simulink model "rlAgentLCLongLat"  (R2024a)
settings: Solver=VariableStepAuto  StartTime=0.0  StopTime=Tf  FixedStep=1e-3  MaxStep=0.1  RelTol=1e-3
values from neighbouring files (symbols this model uses):
  A = [ ... (first row only)    [rlAgentLCParams.m]
  B = [0 2*Cf/m 0 2*lf*Cf/Iz]'    [rlAgentLCParams.m]
  Cf = 19000    [multiAgentPFCParams.m]    (also in rlAgentLCParams.m = 151000)
  Cr = 33000    [multiAgentPFCParams.m]    (also in rlAgentLCParams.m = 146000)
  Iz = 2875    [multiAgentPFCParams.m]    (also in rlAgentLCParams.m = 1993)
  lf = 1.4    [multiAgentPFCParams.m]    (also in rlAgentLCParams.m = 1.45)
  lr = 1.6    [multiAgentPFCParams.m]    (also in rlAgentLCParams.m = 1.06)
  m = 1600    [multiAgentPFCParams.m]    (also in rlAgentLCParams.m = 1360)
  Qlat = diag([20 50 2000 3000])    [rlAgentLCParams.m]
  Rlat = eye(1)    [rlAgentLCParams.m]
  Ts = 0.1    [rlAgentLCParams.m]
  Vx = 20    [rlAgentLCParams.m]
undefined symbols (not defined in the file or in its folder): Qlong, Rlong
libraries: rllib x2, matrix_library x2
settings Model: Creator=The MathWorks, Inc.  LastModifiedBy=canlab
settings SolverCC: AlgebraicLoopSolver=TrustRegion
settings DataIOCC: SaveOutput=off  SignalLogging=off  DSMLogging=off  SaveTime=off  ReturnWorkspaceOutputs=off
settings DebuggingCC: ParameterPrecisionLossMsg=none  UnconnectedInputMsg=warning  UnconnectedOutputMsg=warning  UnconnectedLineMsg=warning  ArithmeticOperatorsInVariantConditions=warning
settings ModelReferenceCC: EnableRefExpFcnMdlSchedulingChecks=on
settings SFSimCC: SimUseLocalCustomCode=off
settings RTWCC: RTWUseLocalCustomCode=off  GPUComputeCapability=3.5  DLArmComputeVersion=19.05

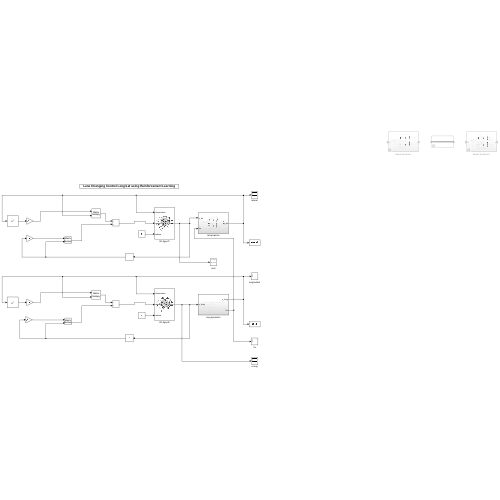
[thumbnail: Simulink's stored preview of the top-level diagram]
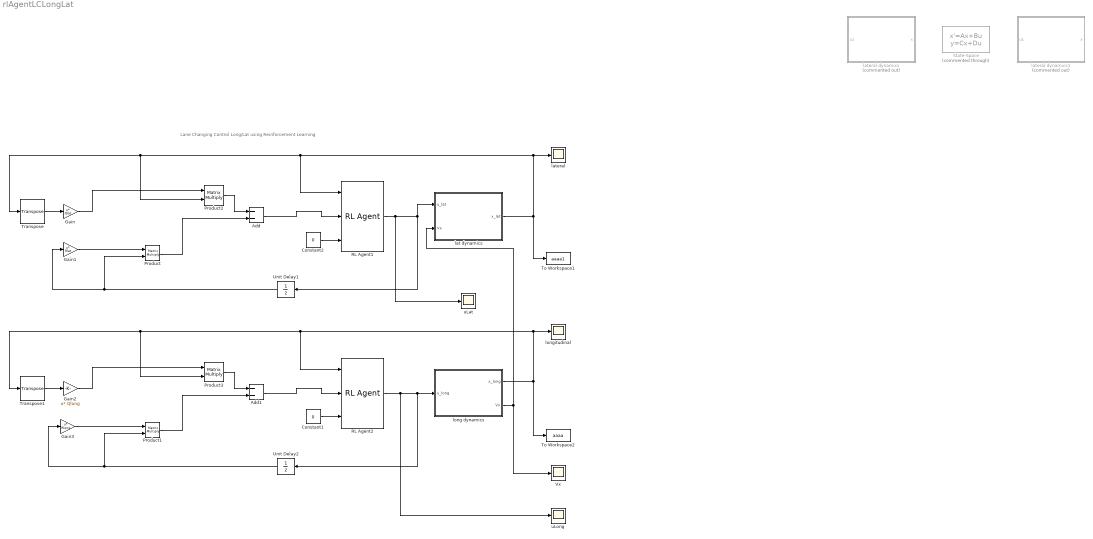
== system rlAgentLCLongLat ==
  note: Lane Changing Control Long/Lat using Reinforcement Learning
  Add : Sum  Inputs=--
  Add1 : Sum  Inputs=--
  Constant1 : Constant  Value=0  SampleTime=Ts
  Constant2 : Constant  Value=0  SampleTime=Ts
  Gain : Gain  Gain=Qlat  Multiplication=Matrix(u*K)
  Gain1 : Gain  Gain=Rlat  Multiplication=Matrix(u*K)
  Gain2 : Gain  Gain=Qlong  Multiplication=Matrix(u*K)
  Gain3 : Gain  Gain=Rlong  Multiplication=Matrix(u*K)
  Product{,1..3} (4 alike) : Product  Multiplication=Matrix(*)
  RL Agent1 : rllib/RL Agent  Agent=agent1  ExternalActionAsInput=off  ProvideLastAction=off  ProvideCumRwd=off  TreatAsDirectFeedthrough=on  UseStrictObservationDataTypes=off
  RL Agent2 : rllib/RL Agent  Agent=agent2  ExternalActionAsInput=off  ProvideLastAction=off  ProvideCumRwd=off  TreatAsDirectFeedthrough=on  UseStrictObservationDataTypes=off
  State-Space : StateSpace  Commented=through  A=A  B=B  C=eye(4)  D=zeros(4,1)  InitialCondition=[1;0;1;0]
  To Workspace1 : ToWorkspace  VariableName=aaaa1  SaveFormat=Timeseries  SampleTime=0.1
  To Workspace2 : ToWorkspace  VariableName=aaaa  SaveFormat=Timeseries  SampleTime=0.1
  Transpose : matrix_library/Transpose
  Transpose1 : matrix_library/Transpose
  Unit Delay1 : UnitDelay  SampleTime=-1  HasFrameUpgradeWarning=on
  Unit Delay2 : UnitDelay  SampleTime=-1  HasFrameUpgradeWarning=on
  Vx : Scope
  lat dynamics : Subsystem
  lateral : Scope
  lateral dynamics : Subsystem  Commented=on
  lateral dynamics1 : Subsystem  Commented=on
  long dynamics : Subsystem
  longitudinal : Scope
  uLat : Scope
  uLong : Scope
  wires:
  Transpose/1 -> Gain/1
  Product2/1 -> Add/1
  Constant2/1 -> RL Agent1/3
  RL Agent1/1 -> uLat/1, lat dynamics/1(u_lat), Unit Delay1/1
  lat dynamics/1(x_lat) -> To Workspace1/1, Transpose/1, Product2/2, RL Agent1/1, lateral/1
  Add/1 -> RL Agent1/2
  Product/1 -> Add/2
  Unit Delay1/1 -> Product/2, Gain1/1
  Gain/1 -> Product2/1
  Gain1/1 -> Product/1
  Unit Delay2/1 -> Gain3/1, Product1/2
  Product1/1 -> Add1/2
  RL Agent2/1 -> uLong/1, long dynamics/1(u_long), Unit Delay2/1
  Product3/1 -> Add1/1
  Add1/1 -> RL Agent2/2
  Gain2/1 -> Product3/1
  long dynamics/1(x_long) -> To Workspace2/1, Transpose1/1, Product3/2, RL Agent2/1, longitudinal/1
  Transpose1/1 -> Gain2/1
  Gain3/1 -> Product1/1
  Constant1/1 -> RL Agent2/3
  long dynamics/2(Vx) -> lat dynamics/2(Vx), Vx/1

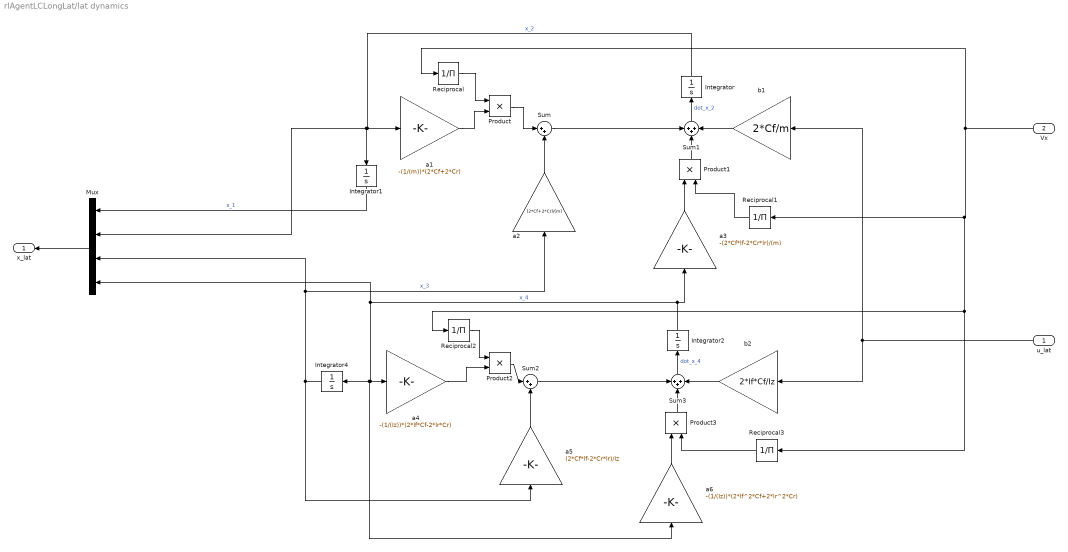
== system rlAgentLCLongLat/lat dynamics ==
  u_lat : Inport
  Vx : Inport  Port=2
  Integrator : Integrator
  Integrator1 : Integrator  InitialCondition=1
  Integrator2 : Integrator
  Integrator4 : Integrator  InitialCondition=1
  Mux : Mux
  Product{,1..3} (4 alike) : Product
  Reciprocal{,1..3} (4 alike) : Product  Inputs=/
  Sum : Sum  Inputs=|++
  Sum1 : Sum  Inputs=+++
  Sum2 : Sum  Inputs=|++
  Sum3 : Sum  Inputs=+++
  a1 : Gain  Gain=-(1/(m))*(2*Cf+2*Cr)
  a2 : Gain  Gain=(2*Cf+2*Cr)/(m)
  a3 : Gain  Gain=-(2*Cf*lf-2*Cr*lr)/(m)
  a4 : Gain  Gain=-(1/(Iz))*(2*lf*Cf-2*lr*Cr)
  a5 : Gain  Gain=(2*Cf*lf-2*Cr*lr)/Iz
  a6 : Gain  Gain=-(1/(Iz))*(2*lf^2*Cf+2*lr^2*Cr)
  b1 : Gain  Gain=2*Cf/m
  b2 : Gain  Gain=2*lf*Cf/Iz
  x_lat : Outport
  wires:
  a3/1 -> Product1/1
  Product1/1 -> Sum1/2
  Sum1/1 -> Integrator/1  "dot_x_2"
  Sum3/1 -> Integrator2/1  "dot_x_4"
  Integrator1/1 -> Mux/1  "x_1"
  u_lat/1 -> b1/1, b2/1
  a2/1 -> Sum/2
  Sum2/1 -> Sum3/1
  Integrator2/1 -> a6/1, Integrator4/1, a4/1, Mux/4, a3/1  "x_4"
  a4/1 -> Product2/2
  Integrator4/1 -> a2/1, Mux/3, a5/1  "x_3"
  Integrator/1 -> Mux/2, Integrator1/1, a1/1  "x_2"
  a5/1 -> Sum2/2
  Product3/1 -> Sum3/2
  Product2/1 -> Sum2/1
  Mux/1 -> x_lat/1
  Reciprocal/1 -> Product/1
  b2/1 -> Sum3/3
  a1/1 -> Product/2
  Vx/1 -> Reciprocal2/1, Reciprocal3/1, Reciprocal1/1, Reciprocal/1
  Reciprocal2/1 -> Product2/1
  Reciprocal1/1 -> Product1/2
  Product/1 -> Sum/1
  Sum/1 -> Sum1/1
  b1/1 -> Sum1/3
  a6/1 -> Product3/1
  Reciprocal3/1 -> Product3/2

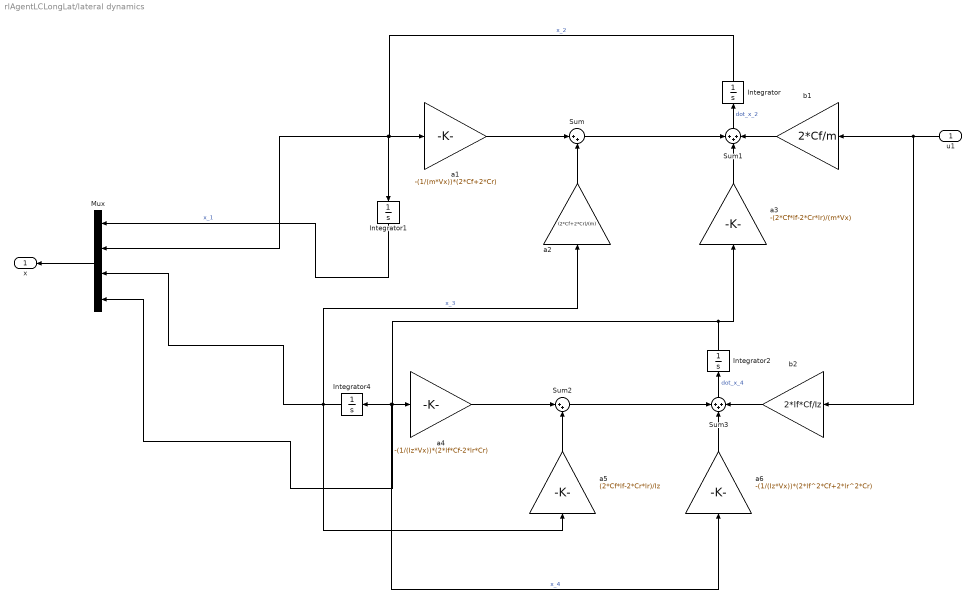
== system rlAgentLCLongLat/lateral dynamics ==
  u1 : Inport
  Integrator : Integrator
  Integrator1 : Integrator  InitialCondition=1
  Integrator2 : Integrator
  Integrator4 : Integrator  InitialCondition=1
  Mux : Mux
  Sum : Sum  Inputs=|++
  Sum1 : Sum  Inputs=+++
  Sum2 : Sum  Inputs=|++
  Sum3 : Sum  Inputs=+++
  a1 : Gain  Gain=-(1/(m*Vx))*(2*Cf+2*Cr)
  a2 : Gain  Gain=(2*Cf+2*Cr)/(m)
  a3 : Gain  Gain=-(2*Cf*lf-2*Cr*lr)/(m*Vx)
  a4 : Gain  Gain=-(1/(Iz*Vx))*(2*lf*Cf-2*lr*Cr)
  a5 : Gain  Gain=(2*Cf*lf-2*Cr*lr)/Iz
  a6 : Gain  Gain=-(1/(Iz*Vx))*(2*lf^2*Cf+2*lr^2*Cr)
  b1 : Gain  Gain=2*Cf/m
  b2 : Gain  Gain=2*lf*Cf/Iz
  x : Outport
  wires:
  Integrator/1 -> Mux/2, Integrator1/1, a1/1  "x_2"
  a6/1 -> Sum3/2
  Sum/1 -> Sum1/1
  a4/1 -> Sum2/1
  Integrator4/1 -> a5/1, a2/1, Mux/3  "x_3"
  a5/1 -> Sum2/2
  Integrator2/1 -> a6/1, Integrator4/1, a4/1, Mux/4, a3/1  "x_4"
  Sum1/1 -> Integrator/1  "dot_x_2"
  Sum2/1 -> Sum3/1
  Sum3/1 -> Integrator2/1  "dot_x_4"
  b2/1 -> Sum3/3
  b1/1 -> Sum1/3
  a2/1 -> Sum/2
  a3/1 -> Sum1/2
  a1/1 -> Sum/1
  u1/1 -> b2/1, b1/1
  Integrator1/1 -> Mux/1  "x_1"
  Mux/1 -> x/1

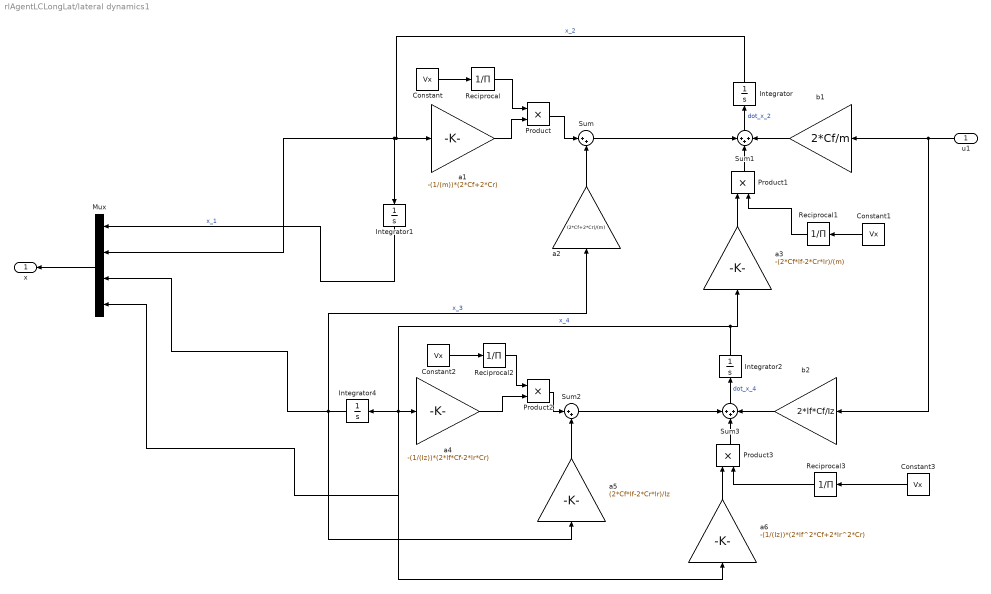
== system rlAgentLCLongLat/lateral dynamics1 ==
  u1 : Inport
  Constant{,1..3} (4 alike) : Constant  Value=Vx
  Integrator : Integrator
  Integrator1 : Integrator  InitialCondition=1
  Integrator2 : Integrator
  Integrator4 : Integrator  InitialCondition=1
  Mux : Mux
  Product{,1..3} (4 alike) : Product
  Reciprocal{,1..3} (4 alike) : Product  Inputs=/
  Sum : Sum  Inputs=|++
  Sum1 : Sum  Inputs=+++
  Sum2 : Sum  Inputs=|++
  Sum3 : Sum  Inputs=+++
  a1 : Gain  Gain=-(1/(m))*(2*Cf+2*Cr)
  a2 : Gain  Gain=(2*Cf+2*Cr)/(m)
  a3 : Gain  Gain=-(2*Cf*lf-2*Cr*lr)/(m)
  a4 : Gain  Gain=-(1/(Iz))*(2*lf*Cf-2*lr*Cr)
  a5 : Gain  Gain=(2*Cf*lf-2*Cr*lr)/Iz
  a6 : Gain  Gain=-(1/(Iz))*(2*lf^2*Cf+2*lr^2*Cr)
  b1 : Gain  Gain=2*Cf/m
  b2 : Gain  Gain=2*lf*Cf/Iz
  x : Outport
  wires:
  Integrator/1 -> Mux/2, Integrator1/1, a1/1  "x_2"
  a6/1 -> Product3/1
  Sum/1 -> Sum1/1
  a4/1 -> Product2/2
  Integrator4/1 -> a5/1, a2/1, Mux/3  "x_3"
  a5/1 -> Sum2/2
  Integrator2/1 -> a6/1, Integrator4/1, a4/1, Mux/4, a3/1  "x_4"
  Sum1/1 -> Integrator/1  "dot_x_2"
  Sum2/1 -> Sum3/1
  Sum3/1 -> Integrator2/1  "dot_x_4"
  b2/1 -> Sum3/3
  b1/1 -> Sum1/3
  a2/1 -> Sum/2
  a3/1 -> Product1/1
  a1/1 -> Product/2
  u1/1 -> b2/1, b1/1
  Integrator1/1 -> Mux/1  "x_1"
  Mux/1 -> x/1
  Reciprocal/1 -> Product/1
  Constant/1 -> Reciprocal/1
  Product/1 -> Sum/1
  Constant1/1 -> Reciprocal1/1
  Reciprocal1/1 -> Product1/2
  Product1/1 -> Sum1/2
  Constant2/1 -> Reciprocal2/1
  Reciprocal2/1 -> Product2/1
  Product2/1 -> Sum2/1
  Constant3/1 -> Reciprocal3/1
  Reciprocal3/1 -> Product3/2
  Product3/1 -> Sum3/2

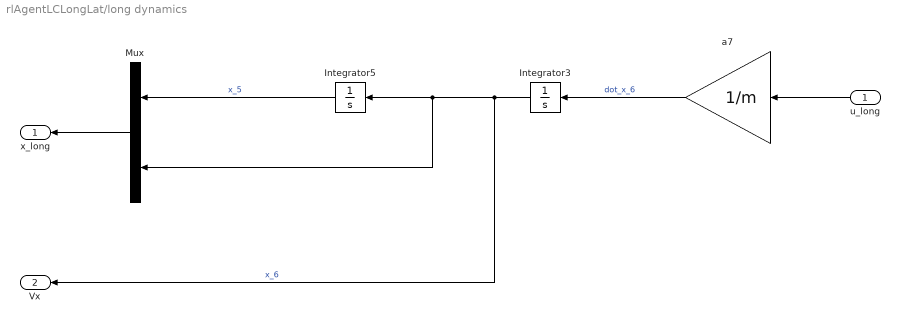
== system rlAgentLCLongLat/long dynamics ==
  u_long : Inport
  Integrator3 : Integrator  InitialCondition=1
  Integrator5 : Integrator  InitialCondition=1
  Mux : Mux  Inputs=2
  a7 : Gain  Gain=1/m
  x_long : Outport
  Vx : Outport  Port=2
  wires:
  u_long/1 -> a7/1
  a7/1 -> Integrator3/1  "dot_x_6"
  Integrator3/1 -> Vx/1, Mux/2, Integrator5/1  "x_6"
  Integrator5/1 -> Mux/1  "x_5"
  Mux/1 -> x_long/1
